simulink model "BF_Drone"  (Simulink 7.4)
settings: Solver=FixedStepDiscrete  StartTime=0.0  StopTime=Tsim  FixedStep=Te  RelTol=1e-3
values from neighbouring files (symbols this model uses):
  g0 = 0.0220    (= 0.022)    [data.m]
  g1 = 0.9970    (= 0.997)    [data.m]
  p0 = 0.0014    [data.m]
  p1 = 0.9994    [data.m]
  p2 = -2.5028e-4    (= -0.00025028)    [data.m]
  p3 = 0.9994    [data.m]
  r0 = 0.0014    [data.m]
  r1 = 0.9996    [data.m]
  r2 = 7.053e-5    (= 7.053e-05)    [data.m]
  r3 = 0.9995    [data.m]
  Te = 5e-3    (= 0.005)    [data.m]
  y0 = 1.3696e-6    (= 1.3696e-06)    [data.m]
  y1 = 0.9937    [data.m]
undefined symbols (not defined in the file or in its folder): DiscIntNeverNeededParam
libraries: simulink x4
CloseFcn:
  | rtwprivate ssgencode ModelCloseRequest BF_Drone
settings Model: Creator=Kevin  LastModifiedBy=jules
settings OptimizationCC: OptimizeModelRefInitCode=on  LifeSpan=1
settings HardwareCC: ProdIntDivRoundTo=Zero  ProdEndianess=LittleEndian  ProdHWDeviceType=Intel->x86/Pentium
settings RTWCC: SystemTargetFile=ert.tlc  GenCodeOnly=on  TemplateMakefile=ert_default_tmf  Description=Real-Time Workshop Embedded Coder  GenerateReport=on  ProcessScript=ert_make_rtw_hook  IncludeHyperlinkInReport=on  LaunchReport=on  TargetLang=C++  GenerateTraceInfo=on  GenerateTraceReport=on  GenerateTraceReportSl=on  GenerateTraceReportSf=on  GenerateTraceReportEml=on  RTWCompilerOptimization=On  CheckMdlBeforeBuild=Warning
settings CodeAppCC: IgnoreCustomStorageClasses=off
settings ERTTargetCC: MultiwordLength=2048  GenerateSampleERTMain=on  SupportNonFinite=off  SupportComplex=off  RootIOFormat=Structure reference  ERTCustomFileTemplate=example_file_process.tlc  ConvertIfToSwitch=off

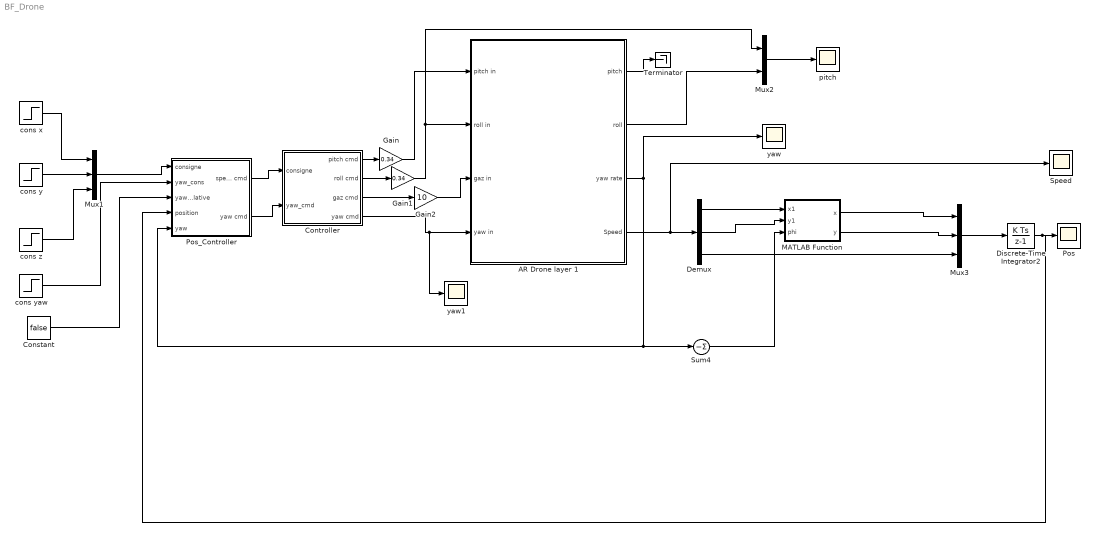
== system BF_Drone ==
  AR Drone layer 1 : Subsystem
  Constant : Constant  Value=false  OutDataTypeMode=boolean  OutDataType=fixdt(1, 16)  OutScaling=2^0  OutDataTypeStr=boolean
  Controller : Subsystem
  Demux : Demux  Outputs=3
  Discrete-Time Integrator2 : DiscreteIntegrator  SampleTime=-1  ICPrevOutput=DiscIntNeverNeededParam  ICPrevScaledInput=DiscIntNeverNeededParam
  Gain : Gain  Gain=0.34  ParameterDataType=fixdt(1, 16)  ParameterScaling=2^0  OutDataType=fixdt(1, 16)  OutScaling=2^0
  Gain1 : Gain  Gain=0.34  ParameterDataType=fixdt(1, 16)  ParameterScaling=2^0  OutDataType=fixdt(1, 16)  OutScaling=2^0
  Gain2 : Gain  Gain=10  ParameterDataType=fixdt(1, 16)  ParameterScaling=2^0  OutDataType=fixdt(1, 16)  OutScaling=2^0
  MATLAB Function : Stateflow chart  TreatAsAtomicUnit=on
  Mux1 : Mux  Inputs=3
  Mux2 : Mux  Inputs=2
  Mux3 : Mux  Inputs=3
  "Pos " : Scope
      settings: TimeRange=60  YMin=3.553487738419619  YMax=3.873487738419619
  Pos_Controller : Subsystem
  Speed : Scope
      settings: TimeRange=60  YMin=3.553487738419619  YMax=3.873487738419619  SaveName=ScopeData2
  Sum4 : Sum  Inputs=|-|
  Terminator : Terminator
  cons x : Step  SampleTime=Te
  cons y : Step  Time=0.1  After=0  SampleTime=Te
  cons yaw : Step  After=0  SampleTime=Te
  cons z : Step  Time=0.1  After=0  SampleTime=Te
  pitch : Scope
  yaw : Scope
      settings: SaveName=ScopeData3
  yaw1 : Scope
      settings: SaveName=ScopeData4
  wires:
  cons x/1 -> Mux1/1
  cons y/1 -> Mux1/2
  cons z/1 -> Mux1/3
  AR Drone layer 1/2(roll) -> Mux2/2
  Controller/1(pitch cmd) -> Gain/1
  Controller/2(roll cmd) -> Gain1/1
  Controller/3(gaz cmd) -> Gain2/1
  Mux2/1 -> pitch/1
  Mux1/1 -> Pos_Controller/1(consigne)
  Pos_Controller/1(speed cmd) -> Controller/1(consigne)
  Controller/4(yaw cmd) -> AR Drone layer 1/4(yaw in), yaw1/1
  Pos_Controller/2(yaw cmd) -> Controller/2(yaw_cmd)
  Discrete-Time Integrator2/1 -> Pos_Controller/4(position), "Pos "/1
  AR Drone layer 1/4(Speed) -> Speed/1, Demux/1
  Mux3/1 -> Discrete-Time Integrator2/1
  Demux/1 -> MATLAB Function/1(x1)
  Demux/2 -> MATLAB Function/2(y1)
  Demux/3 -> Mux3/3
  MATLAB Function/1(x) -> Mux3/1
  MATLAB Function/2(y) -> Mux3/2
  Sum4/1 -> MATLAB Function/3(phi)
  AR Drone layer 1/3(yaw rate) -> yaw/1, Pos_Controller/5(yaw), Sum4/1
  AR Drone layer 1/1(pitch) -> Terminator/1
  cons yaw/1 -> Pos_Controller/2(yaw_cons)
  Gain/1 -> AR Drone layer 1/1(pitch in)
  Gain1/1 -> AR Drone layer 1/2(roll in), Mux2/1
  Gain2/1 -> AR Drone layer 1/3(gaz in)
  Constant/1 -> Pos_Controller/3(yaw_is_relative)

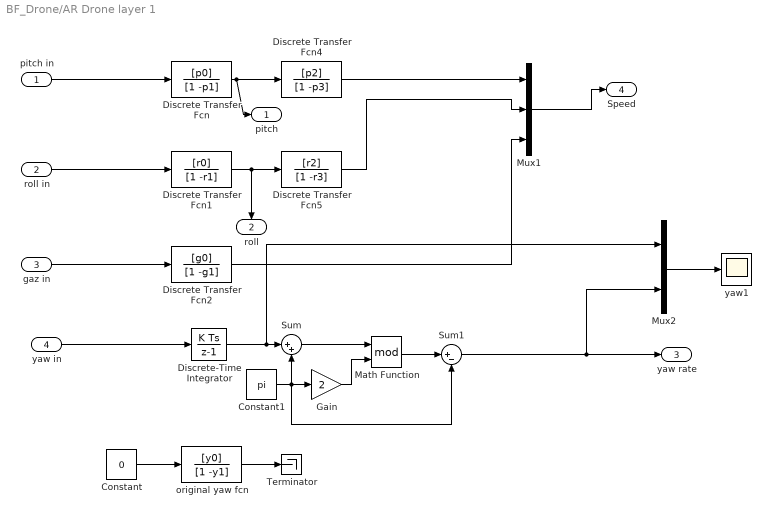
== system BF_Drone/AR Drone layer 1 ==
  pitch in : Inport
  roll in : Inport  Port=2
  gaz in : Inport  Port=3
  yaw in : Inport  Port=4
  Constant : Constant  Value=0  OutDataType=fixdt(1, 16)  OutScaling=2^0
  Constant1 : Constant  Value=pi  OutDataType=fixdt(1, 16)  OutScaling=2^0
  Discrete Transfer Fcn : DiscreteTransferFcn  Numerator=[p0]  Denominator=[1 -p1]  SampleTime=Te
  Discrete Transfer Fcn1 : DiscreteTransferFcn  Numerator=[r0]  Denominator=[1 -r1]  SampleTime=Te
  Discrete Transfer Fcn2 : DiscreteTransferFcn  Numerator=[g0]  Denominator=[1 -g1]  SampleTime=Te
  Discrete Transfer Fcn4 : DiscreteTransferFcn  Numerator=[p2]  Denominator=[1 -p3]  SampleTime=Te
  Discrete Transfer Fcn5 : DiscreteTransferFcn  Numerator=[r2]  Denominator=[1 -r3]  SampleTime=Te
  Discrete-Time Integrator : DiscreteIntegrator  gainval=0.005  SampleTime=Te  OutDataType=fixdt(1, 16)  OutScaling=2^0  ICPrevOutput=DiscIntNeverNeededParam  ICPrevScaledInput=DiscIntNeverNeededParam
  Gain : Gain  Gain=2  ParameterDataType=fixdt(1, 16)  ParameterScaling=2^0  OutDataType=fixdt(1, 16)  OutScaling=2^0
  Math Function : Math  Operator=mod  OutMin=-pi  OutMax=pi  OutDataType=fixdt(1, 16)  OutScaling=2^0  SaturateOnIntegerOverflow=on
  Mux1 : Mux  Inputs=3
  Mux2 : Mux  Inputs=2
  Sum : Sum  Inputs=|++  OutDataType=fixdt(1, 16)  OutScaling=2^0
  Sum1 : Sum  Inputs=|+-  OutDataType=fixdt(1, 16)  OutScaling=2^0
  Terminator : Terminator
  original yaw fcn : DiscreteTransferFcn  Numerator=[y0]  Denominator=[1 -y1]  SampleTime=Te
  yaw1 : Scope
      settings: SaveName=ScopeData5
  pitch : Outport
  roll : Outport  Port=2
  yaw rate : Outport  Port=3
  Speed : Outport  Port=4
  wires:
  Discrete Transfer Fcn1/1 -> Discrete Transfer Fcn5/1, roll/1
  Discrete Transfer Fcn/1 -> Discrete Transfer Fcn4/1, pitch/1
  Discrete Transfer Fcn4/1 -> Mux1/1
  Discrete Transfer Fcn5/1 -> Mux1/2
  Discrete Transfer Fcn2/1 -> Mux1/3
  Discrete-Time Integrator/1 -> Mux2/1, Sum/1
  yaw in/1 -> Discrete-Time Integrator/1
  gaz in/1 -> Discrete Transfer Fcn2/1
  roll in/1 -> Discrete Transfer Fcn1/1
  pitch in/1 -> Discrete Transfer Fcn/1
  Mux1/1 -> Speed/1
  Constant/1 -> original yaw fcn/1
  original yaw fcn/1 -> Terminator/1
  Mux2/1 -> yaw1/1
  Constant1/1 -> Sum/2, Gain/1, Sum1/2
  Sum/1 -> Math Function/1
  Gain/1 -> Math Function/2
  Math Function/1 -> Sum1/1
  Sum1/1 -> yaw rate/1, Mux2/2

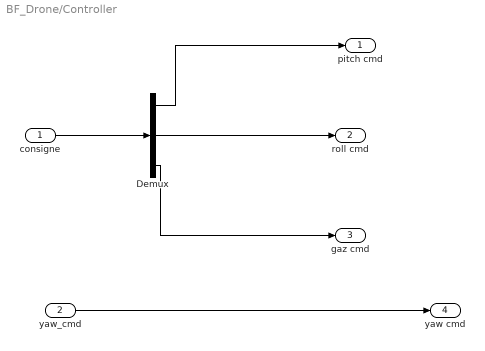
== system BF_Drone/Controller ==
  consigne : Inport
  yaw_cmd : Inport  Port=2
  Demux : Demux  Outputs=3
  pitch cmd : Outport
  roll cmd : Outport  Port=2
  gaz cmd : Outport  Port=3
  yaw cmd : Outport  Port=4
  wires:
  Demux/3 -> gaz cmd/1
  Demux/1 -> pitch cmd/1
  Demux/2 -> roll cmd/1
  yaw_cmd/1 -> yaw cmd/1
  consigne/1 -> Demux/1

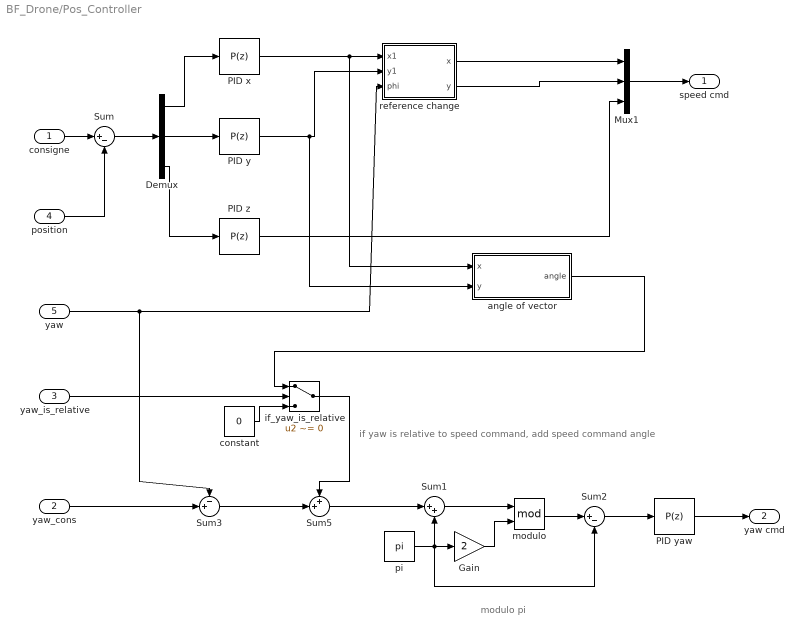
== system BF_Drone/Pos_Controller ==
  note: modulo pi
  note: if yaw is relative to speed command, add speed command angle
  consigne : Inport
  yaw_cons : Inport  Port=2
  yaw_is_relative : Inport  Port=3  DataType=boolean  OutDataTypeStr=boolean
  position : Inport  Port=4  PortDimensions=3
  yaw : Inport  Port=5
  Demux : Demux  Outputs=3
  Gain : Gain  Gain=2  ParameterDataType=fixdt(1, 16)  ParameterScaling=2^0  OutDataType=fixdt(1, 16)  OutScaling=2^0
  Mux1 : Mux  Inputs=3
  PID x : simulink/Continuous/PID Controller  DialogController=pidpack.PIDConfig.pidDDGCreate  DialogControllerArgs=DataTag0  SystemSampleTime=-1  Controller=P  TimeDomain=Discrete-time  SampleTime=Te  IntegratorMethod=Forward Euler  FilterMethod=Forward Euler  Form=Parallel  P=1  I=0.00145262221659031  D=27.5416466320608  N=51.5067222299873  InitialConditionSource=internal  InitialConditionForIntegrator=0  InitialConditionForFilter=0  ExternalReset=none  LimitOutput=on  UpperSaturationLimit=1  LowerSaturationLimit=-1  LinearizeAsGain=off  AntiWindupMode=clamping  Kb=1  TrackingMode=off  Kt=1  PParamMin=[]  PParamMax=[]  IParamMin=[]  IParamMax=[]  DParamMin=[]  DParamMax=[]  NParamMin=[]  NParamMax=[]  KbParamMin=[]  KbParamMax=[]  KtParamMin=[]  KtParamMax=[]  POutMin=[]  POutMax=[]  IOutMin=[]  IOutMax=[]  DOutMin=[]  DOutMax=[]  NOutMin=[]  NOutMax=[]  KbOutMin=[]  KbOutMax=[]  KtOutMin=[]  KtOutMax=[]  IntegratorOutMin=[]  IntegratorOutMax=[]  FilterOutMin=[]  FilterOutMax=[]  SumOutMin=[]  SumOutMax=[]  SumI1OutMin=[]  SumI1OutMax=[]  SumI2OutMin=[]  SumI2OutMax=[]  SumI3OutMin=[]  SumI3OutMax=[]  SumDOutMin=[]  SumDOutMax=[]  SaturationOutMin=[]  SaturationOutMax=[]  IntegratorContinuousStateAttributes=''  IntegratorStateMustResolveToSignalObject=off  IntegratorRTWStateStorageClass=Auto  FilterContinuousStateAttributes=''  FilterStateMustResolveToSignalObject=off  FilterRTWStateStorageClass=Auto
      link override u: SampleTime=SampleTime
  PID y : simulink/Continuous/PID Controller  DialogController=pidpack.PIDConfig.pidDDGCreate  DialogControllerArgs=DataTag1  SystemSampleTime=-1  Controller=P  TimeDomain=Discrete-time  SampleTime=Te  IntegratorMethod=Forward Euler  FilterMethod=Forward Euler  Form=Parallel  P=0.419977099833457  I=0.00145262221659031  D=27.5416466320608  N=51.5067222299873  InitialConditionSource=internal  InitialConditionForIntegrator=0  InitialConditionForFilter=0  ExternalReset=none  LimitOutput=on  UpperSaturationLimit=1  LowerSaturationLimit=-1  LinearizeAsGain=off  AntiWindupMode=clamping  Kb=1  TrackingMode=off  Kt=1  PParamMin=[]  PParamMax=[]  IParamMin=[]  IParamMax=[]  DParamMin=[]  DParamMax=[]  NParamMin=[]  NParamMax=[]  KbParamMin=[]  KbParamMax=[]  KtParamMin=[]  KtParamMax=[]  POutMin=[]  POutMax=[]  IOutMin=[]  IOutMax=[]  DOutMin=[]  DOutMax=[]  NOutMin=[]  NOutMax=[]  KbOutMin=[]  KbOutMax=[]  KtOutMin=[]  KtOutMax=[]  IntegratorOutMin=[]  IntegratorOutMax=[]  FilterOutMin=[]  FilterOutMax=[]  SumOutMin=[]  SumOutMax=[]  SumI1OutMin=[]  SumI1OutMax=[]  SumI2OutMin=[]  SumI2OutMax=[]  SumI3OutMin=[]  SumI3OutMax=[]  SumDOutMin=[]  SumDOutMax=[]  SaturationOutMin=[]  SaturationOutMax=[]  IntegratorContinuousStateAttributes=''  IntegratorStateMustResolveToSignalObject=off  IntegratorRTWStateStorageClass=Auto  FilterContinuousStateAttributes=''  FilterStateMustResolveToSignalObject=off  FilterRTWStateStorageClass=Auto
      link override u: SampleTime=SampleTime
  PID yaw : simulink/Continuous/PID Controller  DialogController=pidpack.PIDConfig.pidDDGCreate  DialogControllerArgs=DataTag2  SystemSampleTime=-1  Controller=P  TimeDomain=Discrete-time  SampleTime=Te  IntegratorMethod=Forward Euler  FilterMethod=Forward Euler  Form=Parallel  P=906.014725413774  I=30.3100567502808  D=-123.70397758102  N=5.3134742355323  InitialConditionSource=internal  InitialConditionForIntegrator=0  InitialConditionForFilter=0  ExternalReset=none  LimitOutput=on  UpperSaturationLimit=1  LowerSaturationLimit=-1  LinearizeAsGain=off  AntiWindupMode=clamping  Kb=1  TrackingMode=off  Kt=1  PParamMin=[]  PParamMax=[]  IParamMin=[]  IParamMax=[]  DParamMin=[]  DParamMax=[]  NParamMin=[]  NParamMax=[]  KbParamMin=[]  KbParamMax=[]  KtParamMin=[]  KtParamMax=[]  POutMin=[]  POutMax=[]  IOutMin=[]  IOutMax=[]  DOutMin=[]  DOutMax=[]  NOutMin=[]  NOutMax=[]  KbOutMin=[]  KbOutMax=[]  KtOutMin=[]  KtOutMax=[]  IntegratorOutMin=[]  IntegratorOutMax=[]  FilterOutMin=[]  FilterOutMax=[]  SumOutMin=[]  SumOutMax=[]  SumI1OutMin=[]  SumI1OutMax=[]  SumI2OutMin=[]  SumI2OutMax=[]  SumI3OutMin=[]  SumI3OutMax=[]  SumDOutMin=[]  SumDOutMax=[]  SaturationOutMin=[]  SaturationOutMax=[]  IntegratorContinuousStateAttributes=''  IntegratorStateMustResolveToSignalObject=off  IntegratorRTWStateStorageClass=Auto  FilterContinuousStateAttributes=''  FilterStateMustResolveToSignalObject=off  FilterRTWStateStorageClass=Auto
      link override u: SampleTime=SampleTime
  PID z : simulink/Continuous/PID Controller  DialogController=pidpack.PIDConfig.pidDDGCreate  DialogControllerArgs=DataTag3  SystemSampleTime=-1  Controller=P  TimeDomain=Discrete-time  SampleTime=Te  IntegratorMethod=Forward Euler  FilterMethod=Forward Euler  Form=Parallel  P=2.49090827957311  I=0.213416531462076  D=2.61797553164598  N=21.853072056216  InitialConditionSource=internal  InitialConditionForIntegrator=0  InitialConditionForFilter=0  ExternalReset=none  LimitOutput=on  UpperSaturationLimit=1  LowerSaturationLimit=-1  LinearizeAsGain=off  AntiWindupMode=clamping  Kb=1  TrackingMode=off  Kt=1  PParamMin=[]  PParamMax=[]  IParamMin=[]  IParamMax=[]  DParamMin=[]  DParamMax=[]  NParamMin=[]  NParamMax=[]  KbParamMin=[]  KbParamMax=[]  KtParamMin=[]  KtParamMax=[]  POutMin=[]  POutMax=[]  IOutMin=[]  IOutMax=[]  DOutMin=[]  DOutMax=[]  NOutMin=[]  NOutMax=[]  KbOutMin=[]  KbOutMax=[]  KtOutMin=[]  KtOutMax=[]  IntegratorOutMin=[]  IntegratorOutMax=[]  FilterOutMin=[]  FilterOutMax=[]  SumOutMin=[]  SumOutMax=[]  SumI1OutMin=[]  SumI1OutMax=[]  SumI2OutMin=[]  SumI2OutMax=[]  SumI3OutMin=[]  SumI3OutMax=[]  SumDOutMin=[]  SumDOutMax=[]  SaturationOutMin=[]  SaturationOutMax=[]  IntegratorContinuousStateAttributes=''  IntegratorStateMustResolveToSignalObject=off  IntegratorRTWStateStorageClass=Auto  FilterContinuousStateAttributes=''  FilterStateMustResolveToSignalObject=off  FilterRTWStateStorageClass=Auto
  Sum : Sum  Inputs=|+-
  Sum1 : Sum  Inputs=|++  OutDataType=fixdt(1, 16)  OutScaling=2^0
  Sum2 : Sum  Inputs=|+-  OutDataType=fixdt(1, 16)  OutScaling=2^0
  Sum3 : Sum  Inputs=-+|
  Sum5 : Sum  Inputs=++|
  angle of vector : Subsystem
  constant : Constant  Value=0  OutDataType=fixdt(1, 16)  OutScaling=2^0
  if_yaw_is_relative : Switch  Criteria=u2 ~= 0  OutDataType=fixdt(1, 16)  OutScaling=2^0
  modulo : Math  Operator=mod  OutputSignalType=real  OutMin=-pi  OutMax=pi  OutDataType=fixdt(1, 16)  OutScaling=2^0  SaturateOnIntegerOverflow=on
  pi : Constant  Value=pi  OutDataType=fixdt(1, 16)  OutScaling=2^0
  reference change : Stateflow chart  TreatAsAtomicUnit=on
  speed cmd : Outport
  yaw cmd : Outport  Port=2
  wires:
  Demux/3 -> PID z/1
  PID z/1 -> Mux1/3
  Demux/1 -> PID x/1
  Demux/2 -> PID y/1
  consigne/1 -> Sum/1
  position/1 -> Sum/2
  Sum/1 -> Demux/1
  Mux1/1 -> speed cmd/1
  yaw/1 -> Sum3/1, reference change/3(phi)
  PID yaw/1 -> yaw cmd/1
  yaw_cons/1 -> Sum3/2
  PID x/1 -> reference change/1(x1), angle of vector/1(x)
  PID y/1 -> reference change/2(y1), angle of vector/2(y)
  reference change/1(x) -> Mux1/1
  reference change/2(y) -> Mux1/2
  pi/1 -> Sum1/2, Gain/1, Sum2/2
  Sum1/1 -> modulo/1
  Gain/1 -> modulo/2
  modulo/1 -> Sum2/1
  Sum2/1 -> PID yaw/1
  yaw_is_relative/1 -> if_yaw_is_relative/2
  Sum5/1 -> Sum1/1
  if_yaw_is_relative/1 -> Sum5/1
  Sum3/1 -> Sum5/2
  constant/1 -> if_yaw_is_relative/3
  angle of vector/1(angle) -> if_yaw_is_relative/1

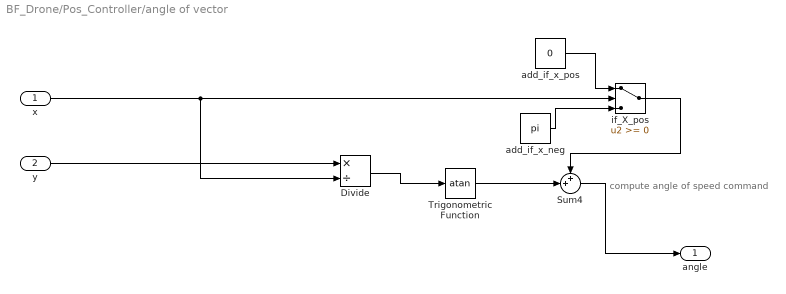
== system BF_Drone/Pos_Controller/angle of vector ==
  note: compute angle of speed command
  x : Inport  OutDataType=fixdt(1, 16)  OutScaling=2^0
  y : Inport  Port=2  OutDataType=fixdt(1, 16)  OutScaling=2^0
  Divide : Product  Inputs=*/  OutDataType=fixdt(1, 16)  OutScaling=2^-10
  Sum4 : Sum  Inputs=++|  OutDataType=fixdt(1, 16)  OutScaling=2^0
  Trigonometric Function : Trigonometry  Operator=atan
  add_if_x_neg : Constant  Value=pi  OutDataType=fixdt(1, 16)  OutScaling=2^0
  add_if_x_pos : Constant  Value=0  OutDataType=fixdt(1, 16)  OutScaling=2^0
  if_X_pos : Switch  OutDataType=fixdt(1, 16)  OutScaling=2^0
  angle : Outport  OutDataType=fixdt(1, 16)  OutScaling=2^0
  wires:
  x/1 -> if_X_pos/2, Divide/2
  y/1 -> Divide/1
  Divide/1 -> Trigonometric Function/1
  Trigonometric Function/1 -> Sum4/2
  add_if_x_neg/1 -> if_X_pos/3
  add_if_x_pos/1 -> if_X_pos/1
  if_X_pos/1 -> Sum4/1
  Sum4/1 -> angle/1

== matlab function Pos_Controller/reference change ==
  data: x1 input double; y1 input double; phi input double; x output double; y output double
function [x,y] = fcn(x1,y1,phi)
%#codegen

[x,y]=changeRep2D(x1,y1,phi);

== matlab function MATLAB Function ==
  data: x1 input double; y1 input double; phi input double; x output double; y output double
function [x,y] = fcn(x1,y1,phi)
%#codegen

[x,y]=changeRep2D(x1,y1,phi);
